simulink model "real_MPC_schema_fixed_v4"  (R2026a)
settings: Solver=ode4  FixedStep=pp.Ts_plant
values from neighbouring files (symbols this model uses):
  params =     [CEM_no_singularity_animation_data.mat]    (also in CEM_singularity_animation_data.mat; test_mpc_singularity_warning_sweep.m = baseParams)
undefined symbols (not defined in the file or in its folder): pp
settings Model: Creator=ryanj  LastModifiedBy=SWP
settings DataIOCC: InspectSignalLogs=on

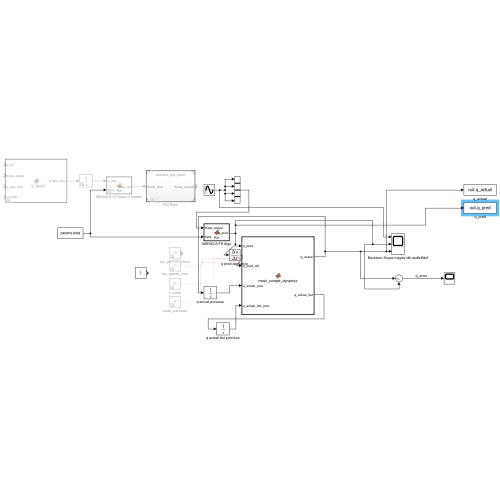
[thumbnail: Simulink's stored preview of the top-level diagram]
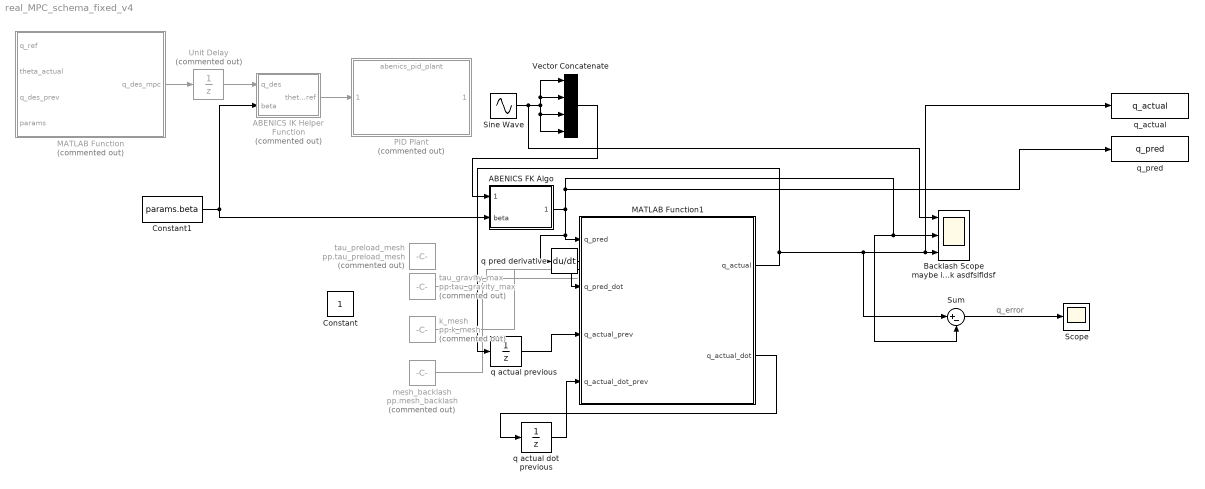
== system real_MPC_schema_fixed_v4 ==
  note: q_error
  ABENICS FK Algo : MATLAB Function  TreatAsAtomicUnit=on
  ABENICS IK Helper Function : MATLAB Function  Commented=on  TreatAsAtomicUnit=on
  Backlash Scope maybe idk asdfslfldsf : Scope  NumInputPorts=3
      settings: Title=Backlash  ActiveDisplayYMinimum=-1.1728275106772379  ActiveDisplayYMaximum=1.7312871987670448
  Constant : Constant
  Constant1 : Constant  Value=params.beta  SampleTime=params.Ts
  MATLAB Function : MATLAB Function  Commented=on  TreatAsAtomicUnit=on
  MATLAB Function1 : MATLAB Function  TreatAsAtomicUnit=on
  PID Plant : ModelReference  Commented=on  ModelNameDialog=abenics_pid_plant  SimulationMode=Normal  ModelReferenceVersion=1.2
  Scope : Scope
      settings: ActiveDisplayYMinimum=-0.060487454138757064  ActiveDisplayYMaximum=0.053081000942398475
  Sine Wave : Sin  SampleTime=0
  Sum : Sum  Inputs=|+-
  Unit Delay : UnitDelay  Commented=on  InitialCondition=[0; 0; 0]  SampleTime=-1
  Vector Concatenate : Concatenate  NumInputs=4
  k_mesh : Constant  Commented=on  Value=pp.k_mesh
  mesh_backlash : Constant  Commented=on  Value=pp.mesh_backlash
  q actual dot previous : UnitDelay  InitialCondition=[0; 0; 0]  SampleTime=pp.Ts_plant
  q actual previous : UnitDelay  InitialCondition=[0; 0; 0]  SampleTime=pp.Ts_plant
  q pred derivative : Derivative
  q_actual : ToWorkspace  VariableName=q_actual  SaveFormat=Timeseries  SampleTime=-1
  q_pred : ToWorkspace  VariableName=q_pred  SaveFormat=Timeseries  SampleTime=-1
  tau_gravity_max : Constant  Commented=on  Value=pp.tau_gravity_max
  tau_preload_mesh : Constant  Commented=on  Value=pp.tau_preload_mesh
  wires:
  Constant1/1 -> ABENICS IK Helper Function/2(beta), ABENICS FK Algo/2(beta)
  MATLAB Function/1(q_des_mpc) -> Unit Delay/1
  Unit Delay/1 -> ABENICS IK Helper Function/1(q_des)
  ABENICS IK Helper Function/1(theta_ref) -> PID Plant/1
  ABENICS FK Algo/1(q_pred) -> Backlash Scope maybe idk asdfslfldsf/2, Sum/2, q_pred/1, q pred derivative/1, MATLAB Function1/1(q_pred)
  tau_gravity_max/1 -> ?
  k_mesh/1 -> ?
  mesh_backlash/1 -> ?
  MATLAB Function1/1(q_actual) -> q_actual/1, Backlash Scope maybe idk asdfslfldsf/3, Sum/1, q actual previous/1
  Sine Wave/1 -> Backlash Scope maybe idk asdfslfldsf/1, Vector Concatenate/2, Vector Concatenate/1, Vector Concatenate/4, Vector Concatenate/3
  Vector Concatenate/1 -> ABENICS FK Algo/1(theta_actual)
  MATLAB Function1/2(q_actual_dot) -> q actual dot previous/1
  q actual previous/1 -> MATLAB Function1/3(q_actual_prev)
  q actual dot previous/1 -> MATLAB Function1/4(q_actual_dot_prev)
  q pred derivative/1 -> MATLAB Function1/2(q_pred_dot)
  Sum/1 -> Scope/1

== matlab function real_MPC_schema_fixed_v4/ABENICS FK Algo ==
  data: theta_actual input size=[4,1]; q_pred output size=[3,1]; beta input
function q_pred = fcn(theta_actual, beta)
%#codegen

params.beta = beta;
q_pred = abenicsFK(theta_actual, params);

end

function [q_pred, info] = abenicsFK(theta_actual, params)
%abenicsFK Analytic 4-input FK for ABENICS orientation prediction.
%
% Input:
%   theta_actual = [theta_rA; theta_pA; theta_rB; theta_pB] in radians
%   params       = ABENICS parameter structure with params.beta
%
% Output:
%   q_pred       = [roll; pitch; yaw] in radians
%   info         = diagnostic structure
%
% Project convention:
%   theta_actual is output-side MP gear angle, not raw motor shaft angle.
%
% Important:
%   This FK uses all four theta values.
%   It builds one CS-gear orientation axis from module A,
%   one CS-gear orientation axis from module B,
%   then uses a cross product to complete the rotation matrix.

    if ~isequal(size(theta_actual), [4, 1])
        error('abenicsFK:thetaSize', ...
              'theta_actual must be [theta_rA; theta_pA; theta_rB; theta_pB].');
    end

    if nargin < 2 || ~isfield(params, 'beta')
        error('abenicsFK:missingBeta', ...
              'params.beta is required.');
    end

    beta = params.beta;

    if ~isscalar(beta)
        error('abenicsFK:betaSize', ...
              'params.beta must be scalar.');
    end

    theta_rA = theta_actual(1);
    theta_pA = theta_actual(2);
    theta_rB = theta_actual(3);
    theta_pB = theta_actual(4);

    % Convert output-side MP gear angles to paper-style chain angles
    theta_A1 = theta_rA;
    theta_A2 = -0.5 * theta_pA;

    theta_B1 = theta_rB;
    theta_B2 = -0.5 * theta_pB;

    % -----------------------------
    % Module A axis contribution
    % -----------------------------
    c1 = [cos(theta_A2);
          sin(theta_A1) * sin(theta_A2);
         -cos(theta_A1) * sin(theta_A2)];

    % -----------------------------
    % Module B axis contribution
    %
    % This is the sign/order-sensitive part.
    % It must be verified by IK -> FK round-trip tests.
    % -----------------------------
    v2_B = [cos(theta_B2);
           -sin(theta_B1) * sin(theta_B2);
            cos(theta_B1) * sin(theta_B2)];

    c2 = localRz(beta) * v2_B;

    % -----------------------------
    % Diagnostics before cleanup
    % -----------------------------
    c1Norm = norm(c1);
    c2Norm = norm(c2);
    rawColumnDot = dot(c1, c2);
    rawCross = cross(c1, c2);
    rawCrossNorm = norm(rawCross);

    % -----------------------------
    % Orthonormalize columns
    %
    % e1 = cleaned first column
    % e2 = cleaned second column, made perpendicular to e1
    % e3 = e1 x e2
    % -----------------------------
    tol = 1e-12;

    if c1Norm < tol
        error('abenicsFK:c1Bad', ...
              'Module A column is near zero.');
    end

    e1 = c1 / c1Norm;

    c2_perp = c2 - dot(e1, c2) * e1;
    c2PerpNorm = norm(c2_perp);

    if c2PerpNorm < tol
        error('abenicsFK:columnsParallel', ...
              'Module A and B columns are nearly parallel. FK orientation is poorly defined.');
    end

    e2 = c2_perp / c2PerpNorm;

    e3 = cross(e1, e2);
    e3 = e3 / norm(e3);

    R_BH = [e1, e2, e3];

    % Convert rotation matrix into [roll; pitch; yaw]
    q_pred = localRotmToXYZEuler(R_BH);

    % -----------------------------
    % Diagnostics
    % -----------------------------
    info = struct();
    info.c1 = c1;
    info.c2 = c2;
    info.e1 = e1;
    info.e2 = e2;
    info.e3 = e3;
    info.R_BH = R_BH;

    info.c1Norm = c1Norm;
    info.c2Norm = c2Norm;
    info.columnDot = rawColumnDot;
    info.crossNorm = rawCrossNorm;
    info.c2PerpNorm = c2PerpNorm;
    info.detR = det(R_BH);

    % Useful singularity-ish clue:
    % small means the two module-defined axes are almost parallel
    info.columnSeparationScore = rawCrossNorm;

    if rawCrossNorm < 1e-6
        warning('abenicsFK:nearParallelColumns', ...
                'Module A and B columns are nearly parallel. This may indicate a singular or poorly conditioned configuration.');
    end

    if ~isequal(size(q_pred), [3, 1])
        error('abenicsFK:qPredSize', ...
              'q_pred must be 3x1.');
    end
end

function R = localRz(theta)
    c = cos(theta);
    s = sin(theta);

    R = [c, -s, 0;
         s,  c, 0;
         0,  0, 1];
end

function x_clamped = localClamp(x, lower, upper)
    x_clamped = min(upper, max(lower, x));
end

function q = localRotmToXYZEuler(R)
% Uses convention:
%   R = Rx(roll) * Ry(pitch) * Rz(yaw)

    tol = 1e-12;

    pitch_arg = localClamp(R(1,3), -1, 1);
    pitch = asin(pitch_arg);

    cp = cos(pitch);

    if abs(cp) > tol
        roll = atan2(-R(2,3), R(3,3));
        yaw  = atan2(-R(1,2), R(1,1));
    else
        roll = 0;
        yaw  = atan2(R(2,1), R(2,2));
    end

    q = [roll;
         pitch;
         yaw];
end

== matlab function real_MPC_schema_fixed_v4/ABENICS IK Helper Function ==
  data: q_des input; theta_ref output; beta input
function theta_ref = fcn(q_des, beta)
%#codegen

params.beta = beta;

theta_ref = abenicsIK(q_des, params);

end

== matlab function real_MPC_schema_fixed_v4/MATLAB Function ==
  data: q_ref input; q_des_mpc output; theta_actual input; q_des_prev input; params input
function q_des_mpc = MPC_Block(q_ref, theta_actual, q_des_prev, params)
%#codegen
% MPC_Block
% This block calls the one-file nonlinear MPC.
%
% Inputs:
%   q_ref        = [roll_ref; pitch_ref; yaw_ref]          3x1
%   theta_actual = [theta_rA; theta_pA; theta_rB; theta_pB] 4x1
%   q_des_prev   = previous MPC output                     3x1
%
% Output:
%   q_des_mpc    = [roll_des; pitch_des; yaw_des]          3x1

    % Force correct vector shapes
    q_ref        = reshape(q_ref,        [3, 1]);
    theta_actual = reshape(theta_actual, [4, 1]);
    q_des_prev   = reshape(q_des_prev,   [3, 1]);

    % Call the full MPC .m file
    q_des_mpc = abenicsOrientationMPC(q_ref, theta_actual, q_des_prev, params);

end

== matlab function real_MPC_schema_fixed_v4/MATLAB Function1 ==
  data: q_pred input size=[3 1]; q_pred_dot input size=[3 1]; q_actual output size=[3 1]; q_actual_prev input size=[3 1]; q_actual_dot_prev input size=[3 1]; q_actual_dot output size=[3 1]; meshContact parameter
function [q_actual, q_actual_dot] = mesh_contact_dynamics(q_pred, q_pred_dot, ...
                    q_actual_prev, q_actual_dot_prev, meshContact)
    Ts = meshContact.Ts;
    half_bl = meshContact.mesh_backlash/2;
    d     = q_actual_prev - q_pred;
    d_dot = q_actual_dot_prev - q_pred_dot;

    % d is a 3x1 [roll; pitch; yaw] vector, so apply the contact
    % law independently to each axis. A vector cannot be used directly
    % as the condition of an if statement in a MATLAB Function block.
    Fc = -meshContact.c_free .* d_dot;

    for i = 1:3
        if d(i) > half_bl(i)
            Fc(i) = -meshContact.k_mesh(i)*(d(i) - half_bl(i)) ...
                    - meshContact.c_contact(i)*d_dot(i);
        elseif d(i) < -half_bl(i)
            Fc(i) = -meshContact.k_mesh(i)*(d(i) + half_bl(i)) ...
                    - meshContact.c_contact(i)*d_dot(i);
        end
    end

    tau_gravity = meshContact.tau_gravity_max .* sin(q_actual_prev);
    net = meshContact.tau_preload_mesh - tau_gravity + Fc;

    q_actual_dot = q_actual_dot_prev + (net ./ meshContact.J_mesh) .* Ts;
    q_actual     = q_actual_prev + q_actual_dot .* Ts;
end
